simulink model "ysw"  (R2014a)
settings: Solver=ode45  StartTime=0.0  StopTime=5  RelTol=1e-3
libraries: simulink x1
settings Model: Creator=Administrator  LastModifiedBy=Administrator

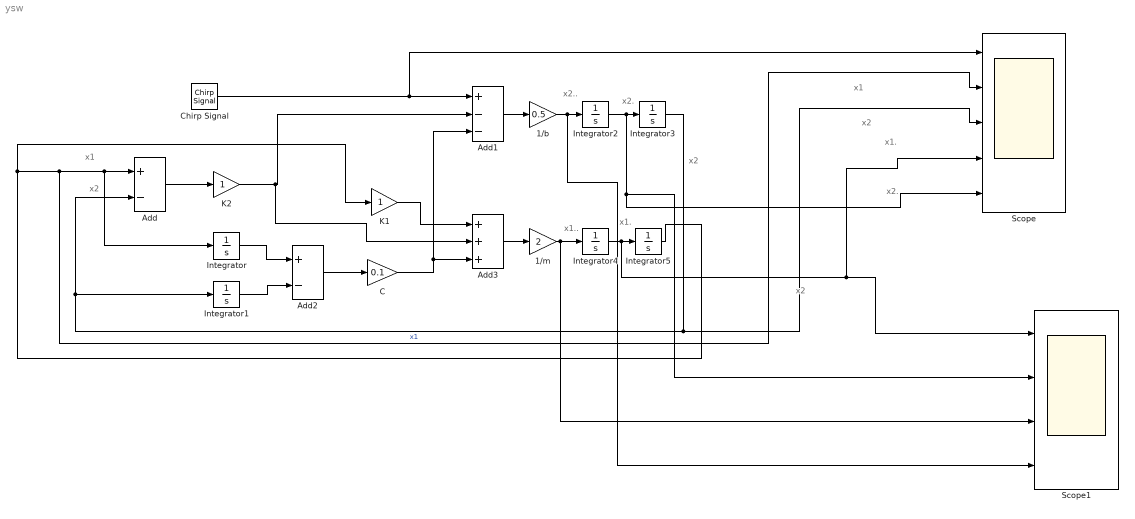
== system ysw ==
  note: x2.
  note: x1.
  note: x2
  note: x1
  note: x2.
  note: x2
  note: x1.
  note: x1..
  note: x2
  note: x2
  note: x1
  note: x2..
  1/b : Gain  Gain=0.5
  1/m : Gain  Gain=2
  Add : Sum  Inputs=+-
  Add1 : Sum  Inputs=+--
  Add2 : Sum  Inputs=+-
  Add3 : Sum  Inputs=+++
  C : Gain  Gain=0.1
  Chirp Signal : simulink/Sources/Chirp Signal  f1=10  T=100  f2=1
  Integrator{,1..5} (6 alike) : Integrator
  K1 : Gain
  K2 : Gain
  Scope : Scope  NumInputPorts=5
      settings: YMin=-5~-5~-5~-5~-5  YMax=5~5~5~5~5
  Scope1 : Scope  NumInputPorts=4
      settings: YMin=-5~-5~-5~-5  YMax=5~5~5~5
  wires:
  Chirp Signal/1 -> Scope/1, Add1/1
  Add/1 -> K2/1
  Add2/1 -> C/1
  Integrator5/1 -> Scope/2, Integrator/1, Add/1, K1/1  "x1"
  Integrator/1 -> Add2/1
  Integrator3/1 -> Add/2, Integrator1/1, Scope/3
  Integrator1/1 -> Add2/2
  K2/1 -> Add3/2, Add1/2
  C/1 -> Add3/3, Add1/3
  Add1/1 -> 1/b/1
  1/b/1 -> Scope1/4, Integrator2/1
  Integrator2/1 -> Scope1/2, Scope/5, Integrator3/1
  K1/1 -> Add3/1
  Add3/1 -> 1/m/1
  Integrator4/1 -> Scope1/1, Scope/4, Integrator5/1
  1/m/1 -> Scope1/3, Integrator4/1
